simulink model "Ass3_SISOopen_NL"  (Simulink 8.1)
settings: Solver=ode45  SolverMode=SingleTasking  StartTime=0.0  StopTime=T  RelTol=1e-3
settings Model: Creator=schuurmans  LastModifiedBy=mpvlaar
settings DataIOCC: ExternalInput=[t, u_in]  LimitDataPoints=off  SaveTime=off
settings OptimizationCC: BlockReduction=off  BooleanDataType=off  InitFltsAndDblsToZero=on
settings DebuggingCC: SaveWithParameterizedLinksMsg=none  SignalResolutionControl=TryResolveAllWithWarning  SolverPrmCheckMsg=none  MultiTaskDSMMsg=warning  MultiTaskCondExecSysMsg=none  FcnCallInpInsideContextMsg=EnableAllAsWarning  StrictBusMsg=None
settings HardwareCC: TargetUnknown=on
settings RTWCC: IncludeERTFirstTime=on
settings GRTTargetCC: TargetFcnLib=ansi_tfl_tmw.mat  ModelReferenceCompliant=off  CompOptLevelCompliant=off  MatFileLogging=off

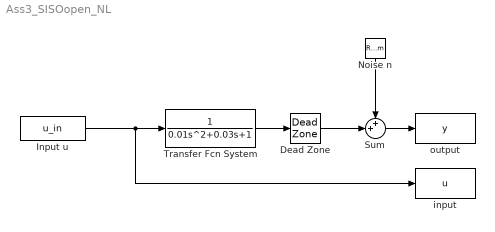
== system Ass3_SISOopen_NL ==
  Dead Zone : DeadZone  LowerValue=-0.3  UpperValue=0.3  SaturateOnIntegerOverflow=on
  Input u : FromWorkspace  VariableName=u_in  SampleTime=0
  Noise n : RandomNumber  Variance=0.1  Seed=61  SampleTime=0
  Sum : Sum  Inputs=++|  SaturateOnIntegerOverflow=on  InputSameDT=on  OutDataTypeStr=Inherit: Same as first input
  Transfer Fcn System : TransferFcn  Denominator=[0.01 0.03 1]
  input : ToWorkspace  VariableName=u  SampleTime=-1
      settings: Description=output
  output : ToWorkspace  VariableName=y  SampleTime=-1
      settings: Description=output
  wires:
  Sum/1 -> output/1
  Input u/1 -> Transfer Fcn System/1, input/1
  Noise n/1 -> Sum/1
  Transfer Fcn System/1 -> Dead Zone/1
  Dead Zone/1 -> Sum/2
